simulink model "MHILSimHWImpl"  (R2024a)
settings: Solver=FixedStepDiscrete  StartTime=0.0  StopTime=2e-4  FixedStep=4e-9  RelTol=1e-3
values from neighbouring files (symbols this model uses):
  cfg = tddbl_model    [HILSimModel.m]
undefined symbols (not defined in the file or in its folder): AXI4, dt, hw, ip, Lite, xc7z020clg400
libraries: hdlBasic x1497, hdlUtilities x3, vmcUtilities x1
(part 11 of 11)

== system MHILSimHWImpl/hilsim_ipcore/proc_domain/slice_2/fb_func/nlf_x ==
  note: Signal should now be normalized
      | to range -1 to 1.
  x : Inport
  presc : Inport  Port=2
  gain : Inport  Port=3
  cfg_select_1 : Inport  Port=4
  cfg_select_2 : Inport  Port=5
  cfg_addr : Inport  Port=6
  cfg_data : Inport  Port=7
  cfg_we : Inport  Port=8
  nlf_switch : Inport  Port=9
  AddSub : hdlBasic/AddSub  mode=Addition  use_carryin=off  use_carryout=off  en=off  latency=1  precision=User Defined  arith_type=Unsigned  n_bits=ip.f_nlf.lut_addr_bits  bin_pt=0  quantization=Truncate  overflow=Wrap  use_behavioral_HDL=off  hw_selection=Fabric  pipelined=off  XmcBlockStatus=1  maskContainerNames=tabcontainer1  block_type=addsub  block_config=sysgen:Addsub_config
  AddSub1 : hdlBasic/AddSub  mode=Subtraction  use_carryin=off  use_carryout=off  en=off  latency=4  precision=User Defined  arith_type="Signed  (2's comp)"  n_bits=dt.slice.sz  bin_pt=dt.slice.bin  quantization=Truncate  overflow=Wrap  use_behavioral_HDL=off  hw_selection=Fabric  pipelined=off  XmcBlockStatus=1  maskContainerNames=tabcontainer1  block_type=addsub  block_config=sysgen:Addsub_config
  LUT_1 : hdlBasic/Dual Port RAM  depth=ip.f_nlf.lut_sz  initVector=cfg.slice1.x_nlf.lut  distributed_mem=Block RAM  init_a=0  init_b=0  rst_a=off  rst_b=off  en_a=off  en_b=off  latency=1  write_mode_A=Read After Write  write_mode_B=Read After Write  explicit_period=[]  period=[]  simulation_type=fast_sim  XmcBlockStatus=1  maskContainerNames=tabcontainer1  block_type=dpram  block_config=sysgen:Dpram_config  optimize=Area
      settings: infoedit=[]
  LUT_2 : hdlBasic/Dual Port RAM  depth=ip.f_nlf.lut_sz  initVector=cfg.slice1.x_nlf.lut  distributed_mem=Block RAM  init_a=0  init_b=0  rst_a=off  rst_b=off  en_a=off  en_b=off  latency=1  write_mode_A=Read After Write  write_mode_B=Read After Write  explicit_period=[]  period=[]  simulation_type=fast_sim  XmcBlockStatus=1  maskContainerNames=tabcontainer1  block_type=dpram  block_config=sysgen:Dpram_config  optimize=Area
      settings: infoedit=[]
  Register{1..4} (4 alike) : hdlBasic/Register  init=0  rst=off  en=off  XmcBlockStatus=1  maskContainerNames=tabcontainer1  block_type=register  block_config=sysgen:Register_config
  Reinterpret : hdlBasic/Reinterpret  force_arith_type=on  arith_type=Unsigned  force_bin_pt=on  bin_pt=0  XmcBlockStatus=1  maskContainerNames=group1  block_type=reinterpret  block_config=sysgen:Reinterpret_config
  add_interpolate : hdlBasic/AddSub  mode=Addition  use_carryin=off  use_carryout=off  en=off  latency=1  precision=User Defined  arith_type="Signed  (2's comp)"  n_bits=dt.slice.sz  bin_pt=dt.slice.bin  quantization=Truncate  overflow=Wrap  use_behavioral_HDL=off  hw_selection=Fabric  pipelined=off  XmcBlockStatus=1  maskContainerNames=tabcontainer1  block_type=addsub  block_config=sysgen:Addsub_config
  addra_mux : hdlBasic/Mux  inputs=2  en=off  latency=1  precision=Full  arith_type=Unsigned  n_bits=16  bin_pt=14  quantization=Truncate  overflow=Wrap  XmcBlockStatus=1  maskContainerNames=tabcontainer1  block_type=mux  block_config=sysgen:Mux_config
  "addra_mux_2 " : hdlBasic/Mux  inputs=2  en=off  latency=1  precision=Full  arith_type=Unsigned  n_bits=16  bin_pt=14  quantization=Truncate  overflow=Wrap  XmcBlockStatus=1  maskContainerNames=tabcontainer1  block_type=mux  block_config=sysgen:Mux_config
  bool_zero_we : hdlBasic/Constant  const=0  gui_display_data_type=Boolean  arith_type=Boolean  n_bits=16  bin_pt=14  preci_type=Single  exp_width=8  frac_width=24  explicit_period=off  period=1  XmcBlockStatus=1  maskContainerNames=tabcontainer1  block_type=constant  block_config=sysgen:Constant_config
  bool_zero_we1 : hdlBasic/Constant  const=0  gui_display_data_type=Boolean  arith_type=Boolean  n_bits=16  bin_pt=14  preci_type=Single  exp_width=8  frac_width=24  explicit_period=off  period=1  XmcBlockStatus=1  maskContainerNames=tabcontainer1  block_type=constant  block_config=sysgen:Constant_config
  bool_zero_wea : hdlBasic/Constant  const=0  gui_display_data_type=Boolean  arith_type=Boolean  n_bits=16  bin_pt=14  preci_type=Single  exp_width=8  frac_width=24  explicit_period=off  period=1  XmcBlockStatus=1  maskContainerNames=tabcontainer1  block_type=constant  block_config=sysgen:Constant_config
  bool_zero_wea_2 : hdlBasic/Constant  const=0  gui_display_data_type=Boolean  arith_type=Boolean  n_bits=16  bin_pt=14  preci_type=Single  exp_width=8  frac_width=24  explicit_period=off  period=1  XmcBlockStatus=1  maskContainerNames=tabcontainer1  block_type=constant  block_config=sysgen:Constant_config
  cast_cutoff_lsbits : hdlBasic/Convert  gui_display_data_type=Fixed-point  arith_type="Signed  (2's comp)"  n_bits=ip.f_nlf.lut_addr_bits  bin_pt=ip.f_nlf.lut_addr_bits-1  float_type=Single  exp_bits=8  fraction_bits=24  quantization=Truncate  overflow=Wrap  en=off  latency=0  pipeline=off  XmcBlockStatus=1  maskContainerNames=group2  block_type=convert  block_config=sysgen:Convert_config  block_width=595  block_height=885
  cast_to_dt/slice : hdlBasic/Convert  gui_display_data_type=Fixed-point  arith_type="Signed  (2's comp)"  n_bits=dt.slice.sz  bin_pt=dt.slice.bin  float_type=Single  exp_bits=8  fraction_bits=24  quantization=Truncate  overflow=Wrap  en=off  latency=0  pipeline=off  XmcBlockStatus=1  maskContainerNames=group2  block_type=convert  block_config=sysgen:Convert_config  block_width=595  block_height=885
  const_1 : hdlBasic/Constant  const=1.0  gui_display_data_type=Fixed-point  arith_type=Unsigned  n_bits=ip.f_nlf.lut_addr_bits  bin_pt=0  preci_type=Single  exp_width=8  frac_width=24  explicit_period=off  period=1  XmcBlockStatus=1  maskContainerNames=tabcontainer1  block_type=constant  block_config=sysgen:Constant_config
  const_1_interp : hdlBasic/Constant  const=1  gui_display_data_type=Fixed-point  arith_type=Signed (2's comp)  n_bits=dt.slice.sz  bin_pt=dt.slice.bin  preci_type=Single  exp_width=8  frac_width=24  explicit_period=off  period=1  XmcBlockStatus=1  maskContainerNames=tabcontainer1  block_type=constant  block_config=sysgen:Constant_config
  cutoff_msbits : hdlBasic/Slice  nbits=dt.slice.sz - ip.f_nlf.lut_addr_bits-1  boolean_output=off  mode=Lower Bit Location + Width  bit1=0  base1=MSB of Input  bit0=0  base0=LSB of Input  XmcBlockStatus=1  maskContainerNames=group1  block_type=slice  block_config=sysgen:Slice_config
  data_a_mux : hdlBasic/Mux  inputs=2  en=off  latency=1  precision=Full  arith_type=Unsigned  n_bits=16  bin_pt=14  quantization=Truncate  overflow=Wrap  XmcBlockStatus=1  maskContainerNames=tabcontainer1  block_type=mux  block_config=sysgen:Mux_config
  data_b_mux : hdlBasic/Mux  inputs=2  en=off  latency=1  precision=Full  arith_type=Unsigned  n_bits=16  bin_pt=14  quantization=Truncate  overflow=Wrap  XmcBlockStatus=1  maskContainerNames=tabcontainer1  block_type=mux  block_config=sysgen:Mux_config
  delay_sync_interpolate : hdlBasic/Delay  rst=off  en=off  latency=4  reg_retiming=off  XmcBlockStatus=1  maskContainerNames=group1  block_type=delay  block_config=sysgen:Delay_config
  dina_mux : hdlBasic/Mux  inputs=2  en=off  latency=1  precision=Full  arith_type=Unsigned  n_bits=16  bin_pt=14  quantization=Truncate  overflow=Wrap  XmcBlockStatus=1  maskContainerNames=tabcontainer1  block_type=mux  block_config=sysgen:Mux_config
  dina_mux_2 : hdlBasic/Mux  inputs=2  en=off  latency=1  precision=Full  arith_type=Unsigned  n_bits=16  bin_pt=14  quantization=Truncate  overflow=Wrap  XmcBlockStatus=1  maskContainerNames=tabcontainer1  block_type=mux  block_config=sysgen:Mux_config
  mult_a : hdlBasic/Mult  precision=User Defined  arith_type="Signed  (2's comp)"  n_bits=dt.slice.sz  bin_pt=dt.slice.bin  quantization=Truncate  overflow=Wrap  en=off  latency=2  opt_float=off  fp_mult_usage=No Usage  use_behavioral_HDL=off  opt=Speed  use_embedded=on  optimum_pipeline=off  pipeline=on  use_rpm=on  placement_style=Triangular  XmcBlockStatus=1  maskContainerNames=group1  block_type=mult  block_config=sysgen:Mult_config  block_width=598  block_height=876
  mult_b : hdlBasic/Mult  precision=User Defined  arith_type="Signed  (2's comp)"  n_bits=dt.slice.sz  bin_pt=dt.slice.bin  quantization=Truncate  overflow=Wrap  en=off  latency=2  opt_float=off  fp_mult_usage=No Usage  use_behavioral_HDL=off  opt=Speed  use_embedded=on  optimum_pipeline=off  pipeline=on  use_rpm=on  placement_style=Triangular  XmcBlockStatus=1  maskContainerNames=group1  block_type=mult  block_config=sysgen:Mult_config  block_width=598  block_height=876
  mult_inp_scale : hdlBasic/Mult  precision=User Defined  arith_type="Signed  (2's comp)"  n_bits=dt.slice.sz  bin_pt=dt.slice.sz - 2  quantization=Truncate  overflow=Wrap  en=off  latency=2  opt_float=off  fp_mult_usage=No Usage  use_behavioral_HDL=off  opt=Speed  use_embedded=on  optimum_pipeline=off  pipeline=on  use_rpm=on  placement_style=Triangular  XmcBlockStatus=1  maskContainerNames=group1  block_type=mult  block_config=sysgen:Mult_config  block_width=598  block_height=876
  mult_out_scale : hdlBasic/Mult  precision=User Defined  arith_type="Signed  (2's comp)"  n_bits=dt.slice.sz  bin_pt=dt.slice.bin  quantization=Truncate  overflow=Wrap  en=off  latency=2  opt_float=off  fp_mult_usage=No Usage  use_behavioral_HDL=off  opt=Speed  use_embedded=on  optimum_pipeline=off  pipeline=on  use_rpm=on  placement_style=Triangular  XmcBlockStatus=1  maskContainerNames=group1  block_type=mult  block_config=sysgen:Mult_config  block_width=598  block_height=876
  reint_sliced : hdlBasic/Reinterpret  force_arith_type=on  arith_type=Unsigned  force_bin_pt=on  bin_pt=dt.slice.sz - ip.f_nlf.lut_addr_bits-1  XmcBlockStatus=1  maskContainerNames=group1  block_type=reinterpret  block_config=sysgen:Reinterpret_config
  wea_mux : hdlBasic/Mux  inputs=2  en=off  latency=1  precision=Full  arith_type=Unsigned  n_bits=16  bin_pt=14  quantization=Truncate  overflow=Wrap  XmcBlockStatus=1  maskContainerNames=tabcontainer1  block_type=mux  block_config=sysgen:Mux_config
  wea_mux_2 : hdlBasic/Mux  inputs=2  en=off  latency=1  precision=Full  arith_type=Unsigned  n_bits=16  bin_pt=14  quantization=Truncate  overflow=Wrap  XmcBlockStatus=1  maskContainerNames=tabcontainer1  block_type=mux  block_config=sysgen:Mux_config
  zero_nlf_datatype : hdlBasic/Constant  const=0  gui_display_data_type=Fixed-point  arith_type=Signed (2's comp)  n_bits=dt.nlf.sz  bin_pt=dt.nlf.bin  preci_type=Single  exp_width=8  frac_width=24  explicit_period=off  period=1  XmcBlockStatus=1  maskContainerNames=tabcontainer1  block_type=constant  block_config=sysgen:Constant_config
  zero_nlf_datatype1 : hdlBasic/Constant  const=0  gui_display_data_type=Fixed-point  arith_type=Signed (2's comp)  n_bits=dt.nlf.sz  bin_pt=dt.nlf.bin  preci_type=Single  exp_width=8  frac_width=24  explicit_period=off  period=1  XmcBlockStatus=1  maskContainerNames=tabcontainer1  block_type=constant  block_config=sysgen:Constant_config
  zero_nlf_dina : hdlBasic/Constant  const=0  gui_display_data_type=Fixed-point  arith_type=Signed (2's comp)  n_bits=dt.nlf.sz  bin_pt=dt.nlf.bin  preci_type=Single  exp_width=8  frac_width=24  explicit_period=off  period=1  XmcBlockStatus=1  maskContainerNames=tabcontainer1  block_type=constant  block_config=sysgen:Constant_config
  zero_nlf_dina_2 : hdlBasic/Constant  const=0  gui_display_data_type=Fixed-point  arith_type=Signed (2's comp)  n_bits=dt.nlf.sz  bin_pt=dt.nlf.bin  preci_type=Single  exp_width=8  frac_width=24  explicit_period=off  period=1  XmcBlockStatus=1  maskContainerNames=tabcontainer1  block_type=constant  block_config=sysgen:Constant_config
  f(x) : Outport
  wires:
  x/1 -> mult_inp_scale/1
  presc/1 -> mult_inp_scale/2
  cast_cutoff_lsbits/1 -> Reinterpret/1
  Reinterpret/1 -> "addra_mux_2 "/2, addra_mux/2, AddSub/1
  const_1/1 -> AddSub/2
  AddSub/1 -> LUT_2/4, LUT_1/4
  bool_zero_we/1 -> LUT_1/6
  zero_nlf_datatype/1 -> LUT_1/5
  mult_inp_scale/1 -> cast_cutoff_lsbits/1, cutoff_msbits/1
  cutoff_msbits/1 -> reint_sliced/1
  reint_sliced/1 -> cast_to_dt/slice/1
  cast_to_dt/slice/1 -> AddSub1/2, delay_sync_interpolate/1
  const_1_interp/1 -> AddSub1/1
  delay_sync_interpolate/1 -> mult_b/2
  AddSub1/1 -> mult_a/2
  mult_a/1 -> add_interpolate/1
  mult_b/1 -> add_interpolate/2
  gain/1 -> mult_out_scale/2
  mult_out_scale/1 -> f(x)/1
  dina_mux/1 -> LUT_1/2
  addra_mux/1 -> LUT_1/1
  wea_mux/1 -> LUT_1/3
  bool_zero_wea/1 -> wea_mux/2
  zero_nlf_dina/1 -> dina_mux/2
  cfg_select_1/1 -> wea_mux/1, dina_mux/1, addra_mux/1
  cfg_addr/1 -> "addra_mux_2 "/3, addra_mux/3
  cfg_we/1 -> wea_mux_2/3, wea_mux/3
  add_interpolate/1 -> mult_out_scale/1
  wea_mux_2/1 -> LUT_2/3
  dina_mux_2/1 -> LUT_2/2
  bool_zero_wea_2/1 -> wea_mux_2/2
  cfg_select_2/1 -> wea_mux_2/1, dina_mux_2/1, "addra_mux_2 "/1
  zero_nlf_dina_2/1 -> dina_mux_2/2
  "addra_mux_2 "/1 -> LUT_2/1
  zero_nlf_datatype1/1 -> LUT_2/5
  bool_zero_we1/1 -> LUT_2/6
  cfg_data/1 -> dina_mux_2/3, dina_mux/3
  LUT_1/1 -> Register3/1
  LUT_2/1 -> Register1/1
  data_a_mux/1 -> mult_a/1
  data_b_mux/1 -> mult_b/1
  LUT_1/2 -> Register2/1
  LUT_2/2 -> Register4/1
  nlf_switch/1 -> data_b_mux/1, data_a_mux/1
  Register3/1 -> data_a_mux/2
  Register1/1 -> data_a_mux/3
  Register2/1 -> data_b_mux/2
  Register4/1 -> data_b_mux/3

== system MHILSimHWImpl/hilsim_ipcore/proc_domain/slice_2/fb_func/nlf_xd ==
  note: Signal should now be normalized
      | to range -1 to 1.
  x : Inport
  presc : Inport  Port=2
  gain : Inport  Port=3
  cfg_select_1 : Inport  Port=4
  cfg_select_2 : Inport  Port=5
  cfg_addr : Inport  Port=6
  cfg_data : Inport  Port=7
  cfg_we : Inport  Port=8
  nlf_switch : Inport  Port=9
  AddSub : hdlBasic/AddSub  mode=Addition  use_carryin=off  use_carryout=off  en=off  latency=1  precision=User Defined  arith_type=Unsigned  n_bits=ip.f_nlf.lut_addr_bits  bin_pt=0  quantization=Truncate  overflow=Wrap  use_behavioral_HDL=off  hw_selection=Fabric  pipelined=off  XmcBlockStatus=1  maskContainerNames=tabcontainer1  block_type=addsub  block_config=sysgen:Addsub_config
  AddSub1 : hdlBasic/AddSub  mode=Subtraction  use_carryin=off  use_carryout=off  en=off  latency=4  precision=User Defined  arith_type="Signed  (2's comp)"  n_bits=dt.slice.sz  bin_pt=dt.slice.bin  quantization=Truncate  overflow=Wrap  use_behavioral_HDL=off  hw_selection=Fabric  pipelined=off  XmcBlockStatus=1  maskContainerNames=tabcontainer1  block_type=addsub  block_config=sysgen:Addsub_config
  LUT_1 : hdlBasic/Dual Port RAM  depth=ip.f_nlf.lut_sz  initVector=cfg.slice1.xd_nlf.lut  distributed_mem=Block RAM  init_a=0  init_b=0  rst_a=off  rst_b=off  en_a=off  en_b=off  latency=1  write_mode_A=Read After Write  write_mode_B=Read After Write  explicit_period=[]  period=[]  simulation_type=fast_sim  XmcBlockStatus=1  maskContainerNames=tabcontainer1  block_type=dpram  block_config=sysgen:Dpram_config  optimize=Area
      settings: infoedit=[]
  LUT_2 : hdlBasic/Dual Port RAM  depth=ip.f_nlf.lut_sz  initVector=cfg.slice1.xd_nlf.lut  distributed_mem=Block RAM  init_a=0  init_b=0  rst_a=off  rst_b=off  en_a=off  en_b=off  latency=1  write_mode_A=Read After Write  write_mode_B=Read After Write  explicit_period=[]  period=[]  simulation_type=fast_sim  XmcBlockStatus=1  maskContainerNames=tabcontainer1  block_type=dpram  block_config=sysgen:Dpram_config  optimize=Area
      settings: infoedit=[]
  Register{1..4} (4 alike) : hdlBasic/Register  init=0  rst=off  en=off  XmcBlockStatus=1  maskContainerNames=tabcontainer1  block_type=register  block_config=sysgen:Register_config
  Reinterpret : hdlBasic/Reinterpret  force_arith_type=on  arith_type=Unsigned  force_bin_pt=on  bin_pt=0  XmcBlockStatus=1  maskContainerNames=group1  block_type=reinterpret  block_config=sysgen:Reinterpret_config
  add_interpolate : hdlBasic/AddSub  mode=Addition  use_carryin=off  use_carryout=off  en=off  latency=1  precision=User Defined  arith_type="Signed  (2's comp)"  n_bits=dt.slice.sz  bin_pt=dt.slice.bin  quantization=Truncate  overflow=Wrap  use_behavioral_HDL=off  hw_selection=Fabric  pipelined=off  XmcBlockStatus=1  maskContainerNames=tabcontainer1  block_type=addsub  block_config=sysgen:Addsub_config
  addra_mux : hdlBasic/Mux  inputs=2  en=off  latency=1  precision=Full  arith_type=Unsigned  n_bits=16  bin_pt=14  quantization=Truncate  overflow=Wrap  XmcBlockStatus=1  maskContainerNames=tabcontainer1  block_type=mux  block_config=sysgen:Mux_config
  "addra_mux_2 " : hdlBasic/Mux  inputs=2  en=off  latency=1  precision=Full  arith_type=Unsigned  n_bits=16  bin_pt=14  quantization=Truncate  overflow=Wrap  XmcBlockStatus=1  maskContainerNames=tabcontainer1  block_type=mux  block_config=sysgen:Mux_config
  bool_zero_we : hdlBasic/Constant  const=0  gui_display_data_type=Boolean  arith_type=Boolean  n_bits=16  bin_pt=14  preci_type=Single  exp_width=8  frac_width=24  explicit_period=off  period=1  XmcBlockStatus=1  maskContainerNames=tabcontainer1  block_type=constant  block_config=sysgen:Constant_config
  bool_zero_we1 : hdlBasic/Constant  const=0  gui_display_data_type=Boolean  arith_type=Boolean  n_bits=16  bin_pt=14  preci_type=Single  exp_width=8  frac_width=24  explicit_period=off  period=1  XmcBlockStatus=1  maskContainerNames=tabcontainer1  block_type=constant  block_config=sysgen:Constant_config
  bool_zero_wea : hdlBasic/Constant  const=0  gui_display_data_type=Boolean  arith_type=Boolean  n_bits=16  bin_pt=14  preci_type=Single  exp_width=8  frac_width=24  explicit_period=off  period=1  XmcBlockStatus=1  maskContainerNames=tabcontainer1  block_type=constant  block_config=sysgen:Constant_config
  bool_zero_wea_2 : hdlBasic/Constant  const=0  gui_display_data_type=Boolean  arith_type=Boolean  n_bits=16  bin_pt=14  preci_type=Single  exp_width=8  frac_width=24  explicit_period=off  period=1  XmcBlockStatus=1  maskContainerNames=tabcontainer1  block_type=constant  block_config=sysgen:Constant_config
  cast_cutoff_lsbits : hdlBasic/Convert  gui_display_data_type=Fixed-point  arith_type="Signed  (2's comp)"  n_bits=ip.f_nlf.lut_addr_bits  bin_pt=ip.f_nlf.lut_addr_bits-1  float_type=Single  exp_bits=8  fraction_bits=24  quantization=Truncate  overflow=Wrap  en=off  latency=0  pipeline=off  XmcBlockStatus=1  maskContainerNames=group2  block_type=convert  block_config=sysgen:Convert_config  block_width=595  block_height=885
  cast_to_dt/slice : hdlBasic/Convert  gui_display_data_type=Fixed-point  arith_type="Signed  (2's comp)"  n_bits=dt.slice.sz  bin_pt=dt.slice.bin  float_type=Single  exp_bits=8  fraction_bits=24  quantization=Truncate  overflow=Wrap  en=off  latency=0  pipeline=off  XmcBlockStatus=1  maskContainerNames=group2  block_type=convert  block_config=sysgen:Convert_config  block_width=595  block_height=885
  const_1 : hdlBasic/Constant  const=1.0  gui_display_data_type=Fixed-point  arith_type=Unsigned  n_bits=ip.f_nlf.lut_addr_bits  bin_pt=0  preci_type=Single  exp_width=8  frac_width=24  explicit_period=off  period=1  XmcBlockStatus=1  maskContainerNames=tabcontainer1  block_type=constant  block_config=sysgen:Constant_config
  const_1_interp : hdlBasic/Constant  const=1  gui_display_data_type=Fixed-point  arith_type=Signed (2's comp)  n_bits=dt.slice.sz  bin_pt=dt.slice.bin  preci_type=Single  exp_width=8  frac_width=24  explicit_period=off  period=1  XmcBlockStatus=1  maskContainerNames=tabcontainer1  block_type=constant  block_config=sysgen:Constant_config
  cutoff_msbits : hdlBasic/Slice  nbits=dt.slice.sz - ip.f_nlf.lut_addr_bits-1  boolean_output=off  mode=Lower Bit Location + Width  bit1=0  base1=MSB of Input  bit0=0  base0=LSB of Input  XmcBlockStatus=1  maskContainerNames=group1  block_type=slice  block_config=sysgen:Slice_config
  data_a_mux : hdlBasic/Mux  inputs=2  en=off  latency=1  precision=Full  arith_type=Unsigned  n_bits=16  bin_pt=14  quantization=Truncate  overflow=Wrap  XmcBlockStatus=1  maskContainerNames=tabcontainer1  block_type=mux  block_config=sysgen:Mux_config
  data_b_mux : hdlBasic/Mux  inputs=2  en=off  latency=1  precision=Full  arith_type=Unsigned  n_bits=16  bin_pt=14  quantization=Truncate  overflow=Wrap  XmcBlockStatus=1  maskContainerNames=tabcontainer1  block_type=mux  block_config=sysgen:Mux_config
  delay_sync_interpolate : hdlBasic/Delay  rst=off  en=off  latency=4  reg_retiming=off  XmcBlockStatus=1  maskContainerNames=group1  block_type=delay  block_config=sysgen:Delay_config
  dina_mux : hdlBasic/Mux  inputs=2  en=off  latency=1  precision=Full  arith_type=Unsigned  n_bits=16  bin_pt=14  quantization=Truncate  overflow=Wrap  XmcBlockStatus=1  maskContainerNames=tabcontainer1  block_type=mux  block_config=sysgen:Mux_config
  dina_mux_2 : hdlBasic/Mux  inputs=2  en=off  latency=1  precision=Full  arith_type=Unsigned  n_bits=16  bin_pt=14  quantization=Truncate  overflow=Wrap  XmcBlockStatus=1  maskContainerNames=tabcontainer1  block_type=mux  block_config=sysgen:Mux_config
  mult_a : hdlBasic/Mult  precision=User Defined  arith_type="Signed  (2's comp)"  n_bits=dt.slice.sz  bin_pt=dt.slice.bin  quantization=Truncate  overflow=Wrap  en=off  latency=2  opt_float=off  fp_mult_usage=No Usage  use_behavioral_HDL=off  opt=Speed  use_embedded=on  optimum_pipeline=off  pipeline=on  use_rpm=on  placement_style=Triangular  XmcBlockStatus=1  maskContainerNames=group1  block_type=mult  block_config=sysgen:Mult_config  block_width=598  block_height=876
  mult_b : hdlBasic/Mult  precision=User Defined  arith_type="Signed  (2's comp)"  n_bits=dt.slice.sz  bin_pt=dt.slice.bin  quantization=Truncate  overflow=Wrap  en=off  latency=2  opt_float=off  fp_mult_usage=No Usage  use_behavioral_HDL=off  opt=Speed  use_embedded=on  optimum_pipeline=off  pipeline=on  use_rpm=on  placement_style=Triangular  XmcBlockStatus=1  maskContainerNames=group1  block_type=mult  block_config=sysgen:Mult_config  block_width=598  block_height=876
  mult_inp_scale : hdlBasic/Mult  precision=User Defined  arith_type="Signed  (2's comp)"  n_bits=dt.slice.sz  bin_pt=dt.slice.sz - 2  quantization=Truncate  overflow=Wrap  en=off  latency=2  opt_float=off  fp_mult_usage=No Usage  use_behavioral_HDL=off  opt=Speed  use_embedded=on  optimum_pipeline=off  pipeline=on  use_rpm=on  placement_style=Triangular  XmcBlockStatus=1  maskContainerNames=group1  block_type=mult  block_config=sysgen:Mult_config  block_width=598  block_height=876
  mult_out_scale : hdlBasic/Mult  precision=User Defined  arith_type="Signed  (2's comp)"  n_bits=dt.slice.sz  bin_pt=dt.slice.bin  quantization=Truncate  overflow=Wrap  en=off  latency=2  opt_float=off  fp_mult_usage=No Usage  use_behavioral_HDL=off  opt=Speed  use_embedded=on  optimum_pipeline=off  pipeline=on  use_rpm=on  placement_style=Triangular  XmcBlockStatus=1  maskContainerNames=group1  block_type=mult  block_config=sysgen:Mult_config  block_width=598  block_height=876
  reint_sliced : hdlBasic/Reinterpret  force_arith_type=on  arith_type=Unsigned  force_bin_pt=on  bin_pt=dt.slice.sz - ip.f_nlf.lut_addr_bits-1  XmcBlockStatus=1  maskContainerNames=group1  block_type=reinterpret  block_config=sysgen:Reinterpret_config
  wea_mux : hdlBasic/Mux  inputs=2  en=off  latency=1  precision=Full  arith_type=Unsigned  n_bits=16  bin_pt=14  quantization=Truncate  overflow=Wrap  XmcBlockStatus=1  maskContainerNames=tabcontainer1  block_type=mux  block_config=sysgen:Mux_config
  wea_mux_2 : hdlBasic/Mux  inputs=2  en=off  latency=1  precision=Full  arith_type=Unsigned  n_bits=16  bin_pt=14  quantization=Truncate  overflow=Wrap  XmcBlockStatus=1  maskContainerNames=tabcontainer1  block_type=mux  block_config=sysgen:Mux_config
  zero_nlf_datatype : hdlBasic/Constant  const=0  gui_display_data_type=Fixed-point  arith_type=Signed (2's comp)  n_bits=dt.nlf.sz  bin_pt=dt.nlf.bin  preci_type=Single  exp_width=8  frac_width=24  explicit_period=off  period=1  XmcBlockStatus=1  maskContainerNames=tabcontainer1  block_type=constant  block_config=sysgen:Constant_config
  zero_nlf_datatype1 : hdlBasic/Constant  const=0  gui_display_data_type=Fixed-point  arith_type=Signed (2's comp)  n_bits=dt.nlf.sz  bin_pt=dt.nlf.bin  preci_type=Single  exp_width=8  frac_width=24  explicit_period=off  period=1  XmcBlockStatus=1  maskContainerNames=tabcontainer1  block_type=constant  block_config=sysgen:Constant_config
  zero_nlf_dina : hdlBasic/Constant  const=0  gui_display_data_type=Fixed-point  arith_type=Signed (2's comp)  n_bits=dt.nlf.sz  bin_pt=dt.nlf.bin  preci_type=Single  exp_width=8  frac_width=24  explicit_period=off  period=1  XmcBlockStatus=1  maskContainerNames=tabcontainer1  block_type=constant  block_config=sysgen:Constant_config
  zero_nlf_dina_2 : hdlBasic/Constant  const=0  gui_display_data_type=Fixed-point  arith_type=Signed (2's comp)  n_bits=dt.nlf.sz  bin_pt=dt.nlf.bin  preci_type=Single  exp_width=8  frac_width=24  explicit_period=off  period=1  XmcBlockStatus=1  maskContainerNames=tabcontainer1  block_type=constant  block_config=sysgen:Constant_config
  f(x) : Outport
  wires:
  x/1 -> mult_inp_scale/1
  presc/1 -> mult_inp_scale/2
  cast_cutoff_lsbits/1 -> Reinterpret/1
  Reinterpret/1 -> "addra_mux_2 "/2, addra_mux/2, AddSub/1
  const_1/1 -> AddSub/2
  AddSub/1 -> LUT_2/4, LUT_1/4
  bool_zero_we/1 -> LUT_1/6
  zero_nlf_datatype/1 -> LUT_1/5
  mult_inp_scale/1 -> cast_cutoff_lsbits/1, cutoff_msbits/1
  cutoff_msbits/1 -> reint_sliced/1
  reint_sliced/1 -> cast_to_dt/slice/1
  cast_to_dt/slice/1 -> AddSub1/2, delay_sync_interpolate/1
  const_1_interp/1 -> AddSub1/1
  delay_sync_interpolate/1 -> mult_b/2
  AddSub1/1 -> mult_a/2
  mult_a/1 -> add_interpolate/1
  mult_b/1 -> add_interpolate/2
  gain/1 -> mult_out_scale/2
  mult_out_scale/1 -> f(x)/1
  dina_mux/1 -> LUT_1/2
  addra_mux/1 -> LUT_1/1
  wea_mux/1 -> LUT_1/3
  bool_zero_wea/1 -> wea_mux/2
  zero_nlf_dina/1 -> dina_mux/2
  cfg_select_1/1 -> wea_mux/1, dina_mux/1, addra_mux/1
  cfg_addr/1 -> "addra_mux_2 "/3, addra_mux/3
  cfg_we/1 -> wea_mux_2/3, wea_mux/3
  add_interpolate/1 -> mult_out_scale/1
  wea_mux_2/1 -> LUT_2/3
  dina_mux_2/1 -> LUT_2/2
  bool_zero_wea_2/1 -> wea_mux_2/2
  cfg_select_2/1 -> wea_mux_2/1, dina_mux_2/1, "addra_mux_2 "/1
  zero_nlf_dina_2/1 -> dina_mux_2/2
  "addra_mux_2 "/1 -> LUT_2/1
  zero_nlf_datatype1/1 -> LUT_2/5
  bool_zero_we1/1 -> LUT_2/6
  cfg_data/1 -> dina_mux_2/3, dina_mux/3
  LUT_1/1 -> Register2/1
  LUT_2/1 -> Register1/1
  data_a_mux/1 -> mult_a/1
  data_b_mux/1 -> mult_b/1
  LUT_1/2 -> Register3/1
  LUT_2/2 -> Register4/1
  nlf_switch/1 -> data_b_mux/1, data_a_mux/1
  Register2/1 -> data_a_mux/2
  Register1/1 -> data_a_mux/3
  Register3/1 -> data_b_mux/2
  Register4/1 -> data_b_mux/3

== system MHILSimHWImpl/hilsim_ipcore/proc_domain/slice_2/x_psc/barrel_left_shifter ==
  in : Inport
  shift_by : Inport  Port=2
  Mux : hdlBasic/Mux  inputs=2  en=off  latency=1  precision=Full  arith_type=Unsigned  n_bits=16  bin_pt=14  quantization=Truncate  overflow=Wrap  XmcBlockStatus=1  maskContainerNames=tabcontainer1  block_type=mux  block_config=sysgen:Mux_config
  Mux{1..4} (4 alike) : hdlBasic/Mux  inputs=2  en=off  latency=0  precision=Full  arith_type=Unsigned  n_bits=16  bin_pt=14  quantization=Truncate  overflow=Wrap  XmcBlockStatus=1  maskContainerNames=tabcontainer1  block_type=mux  block_config=sysgen:Mux_config
  bit0 : hdlBasic/Slice  nbits=1  boolean_output=on  mode=Lower Bit Location + Width  bit1=0  base1=MSB of Input  bit0=0  base0=LSB of Input  XmcBlockStatus=1  maskContainerNames=group1  block_type=slice  block_config=sysgen:Slice_config
  bit1 : hdlBasic/Slice  nbits=1  boolean_output=on  mode=Lower Bit Location + Width  bit1=0  base1=MSB of Input  bit0=1  base0=LSB of Input  XmcBlockStatus=1  maskContainerNames=group1  block_type=slice  block_config=sysgen:Slice_config
  bit2 : hdlBasic/Slice  nbits=1  boolean_output=on  mode=Lower Bit Location + Width  bit1=0  base1=MSB of Input  bit0=2  base0=LSB of Input  XmcBlockStatus=1  maskContainerNames=group1  block_type=slice  block_config=sysgen:Slice_config
  bit3 : hdlBasic/Slice  nbits=1  boolean_output=on  mode=Lower Bit Location + Width  bit1=0  base1=MSB of Input  bit0=3  base0=LSB of Input  XmcBlockStatus=1  maskContainerNames=group1  block_type=slice  block_config=sysgen:Slice_config
  bit4 : hdlBasic/Slice  nbits=1  boolean_output=on  mode=Lower Bit Location + Width  bit1=0  base1=MSB of Input  bit0=4  base0=LSB of Input  XmcBlockStatus=1  maskContainerNames=group1  block_type=slice  block_config=sysgen:Slice_config
  shift1 : hdlBasic/Scale  scale_factor=1  XmcBlockStatus=1  maskContainerNames=group1  block_type=scale  block_config=sysgen:Scale_config
  shift16 : hdlBasic/Scale  scale_factor=16  XmcBlockStatus=1  maskContainerNames=group1  block_type=scale  block_config=sysgen:Scale_config
  shift2 : hdlBasic/Scale  scale_factor=2  XmcBlockStatus=1  maskContainerNames=group1  block_type=scale  block_config=sysgen:Scale_config
  shift4 : hdlBasic/Scale  scale_factor=4  XmcBlockStatus=1  maskContainerNames=group1  block_type=scale  block_config=sysgen:Scale_config
  shift8 : hdlBasic/Scale  scale_factor=8  XmcBlockStatus=1  maskContainerNames=group1  block_type=scale  block_config=sysgen:Scale_config
  out : Outport
  wires:
  shift_by/1 -> bit4/1, bit3/1, bit2/1, bit1/1, bit0/1
  shift1/1 -> Mux/3
  in/1 -> shift1/1, Mux/2
  bit0/1 -> Mux/1
  Mux/1 -> shift2/1, Mux1/2
  shift2/1 -> Mux1/3
  shift4/1 -> Mux2/3
  Mux1/1 -> shift4/1, Mux2/2
  shift8/1 -> Mux3/3
  Mux2/1 -> shift8/1, Mux3/2
  bit1/1 -> Mux1/1
  bit2/1 -> Mux2/1
  bit3/1 -> Mux3/1
  Mux3/1 -> shift16/1, Mux4/2
  shift16/1 -> Mux4/3
  Mux4/1 -> out/1
  bit4/1 -> Mux4/1

== system MHILSimHWImpl/hilsim_ipcore/proc_domain/slice_2/xdot_psc/barrel_left_shifter ==
  in : Inport
  shift_by : Inport  Port=2
  Mux : hdlBasic/Mux  inputs=2  en=off  latency=1  precision=Full  arith_type=Unsigned  n_bits=16  bin_pt=14  quantization=Truncate  overflow=Wrap  XmcBlockStatus=1  maskContainerNames=tabcontainer1  block_type=mux  block_config=sysgen:Mux_config
  Mux{1..4} (4 alike) : hdlBasic/Mux  inputs=2  en=off  latency=0  precision=Full  arith_type=Unsigned  n_bits=16  bin_pt=14  quantization=Truncate  overflow=Wrap  XmcBlockStatus=1  maskContainerNames=tabcontainer1  block_type=mux  block_config=sysgen:Mux_config
  bit0 : hdlBasic/Slice  nbits=1  boolean_output=on  mode=Lower Bit Location + Width  bit1=0  base1=MSB of Input  bit0=0  base0=LSB of Input  XmcBlockStatus=1  maskContainerNames=group1  block_type=slice  block_config=sysgen:Slice_config
  bit1 : hdlBasic/Slice  nbits=1  boolean_output=on  mode=Lower Bit Location + Width  bit1=0  base1=MSB of Input  bit0=1  base0=LSB of Input  XmcBlockStatus=1  maskContainerNames=group1  block_type=slice  block_config=sysgen:Slice_config
  bit2 : hdlBasic/Slice  nbits=1  boolean_output=on  mode=Lower Bit Location + Width  bit1=0  base1=MSB of Input  bit0=2  base0=LSB of Input  XmcBlockStatus=1  maskContainerNames=group1  block_type=slice  block_config=sysgen:Slice_config
  bit3 : hdlBasic/Slice  nbits=1  boolean_output=on  mode=Lower Bit Location + Width  bit1=0  base1=MSB of Input  bit0=3  base0=LSB of Input  XmcBlockStatus=1  maskContainerNames=group1  block_type=slice  block_config=sysgen:Slice_config
  bit4 : hdlBasic/Slice  nbits=1  boolean_output=on  mode=Lower Bit Location + Width  bit1=0  base1=MSB of Input  bit0=4  base0=LSB of Input  XmcBlockStatus=1  maskContainerNames=group1  block_type=slice  block_config=sysgen:Slice_config
  shift1 : hdlBasic/Scale  scale_factor=1  XmcBlockStatus=1  maskContainerNames=group1  block_type=scale  block_config=sysgen:Scale_config
  shift16 : hdlBasic/Scale  scale_factor=16  XmcBlockStatus=1  maskContainerNames=group1  block_type=scale  block_config=sysgen:Scale_config
  shift2 : hdlBasic/Scale  scale_factor=2  XmcBlockStatus=1  maskContainerNames=group1  block_type=scale  block_config=sysgen:Scale_config
  shift4 : hdlBasic/Scale  scale_factor=4  XmcBlockStatus=1  maskContainerNames=group1  block_type=scale  block_config=sysgen:Scale_config
  shift8 : hdlBasic/Scale  scale_factor=8  XmcBlockStatus=1  maskContainerNames=group1  block_type=scale  block_config=sysgen:Scale_config
  out : Outport
  wires:
  shift_by/1 -> bit4/1, bit3/1, bit2/1, bit1/1, bit0/1
  shift1/1 -> Mux/3
  in/1 -> shift1/1, Mux/2
  bit0/1 -> Mux/1
  Mux/1 -> shift2/1, Mux1/2
  shift2/1 -> Mux1/3
  shift4/1 -> Mux2/3
  Mux1/1 -> shift4/1, Mux2/2
  shift8/1 -> Mux3/3
  Mux2/1 -> shift8/1, Mux3/2
  bit1/1 -> Mux1/1
  bit2/1 -> Mux2/1
  bit3/1 -> Mux3/1
  Mux3/1 -> shift16/1, Mux4/2
  shift16/1 -> Mux4/3
  Mux4/1 -> out/1
  bit4/1 -> Mux4/1
